simulink model "shared_control"  (R2023b)
settings: Solver=odeN  StartTime=0.0  StopTime=10.0  MaxStep=0.1  MinStep=0.01  RelTol=1e-3
values from neighbouring files (symbols this model uses):
  Bm = B    (= 4.32e-05)    [Admittance_code.m]
  D = 1    [Admittance_code.m]
  J = 2* Jm    (= 1.836e-06)    [Admittance_code.m]
  K = 0.011    [Admittance_code.m]
  Km = K    (= 0.011)    [Admittance_code.m]
  Lw = L    (= 0.00058)    [Admittance_code.m]
  M_inv = 1/J    (= 544662.309368)    [Admittance_code.m]
  Rw = R    (= 1.17)    [Admittance_code.m]
settings Model: Creator=sayeholoumi  LastModifiedBy=sayeholoumi

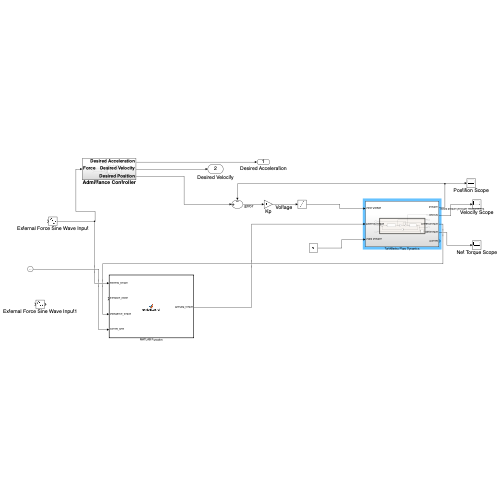
[thumbnail: Simulink's stored preview of the top-level diagram]
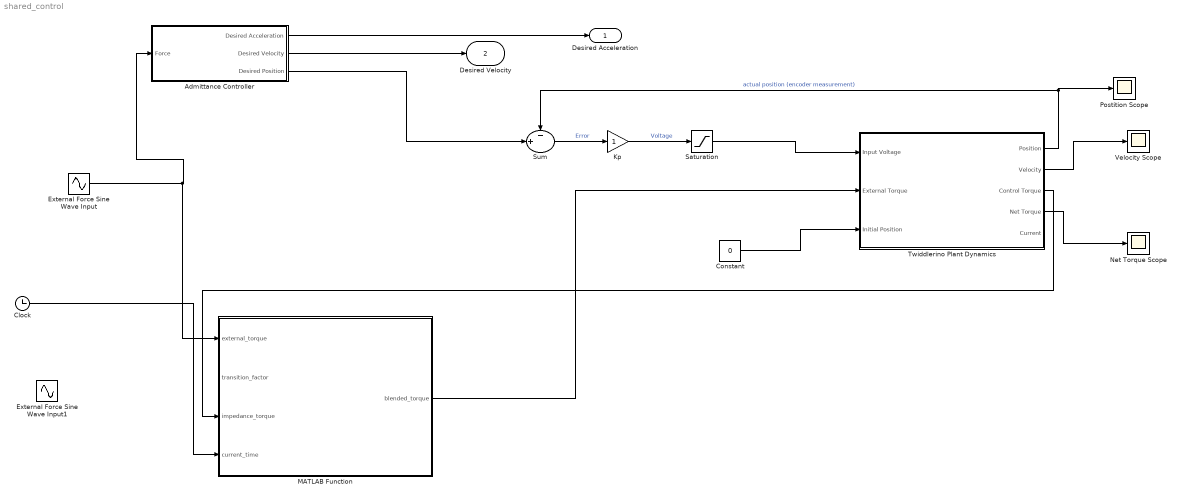
== system shared_control ==
  Admittance Controller : Subsystem
  Clock : Clock
  Constant : Constant  Value=0
  External Force Sine Wave Input : Sin  TimeSource=Use external signal  SampleTime=0
  External Force Sine Wave Input1 : Sin  TimeSource=Use external signal  SampleTime=0
  Kp : Gain
  MATLAB Function : MATLAB Function  TreatAsAtomicUnit=on
  Net Torque Scope : Scope
  Postition Scope : Scope
  Saturation : Saturate  UpperLimit=12  LowerLimit=-12
  Sum : Sum  Inputs=-+|
  Twiddlerino Plant Dynamics : Subsystem
  Velocity Scope : Scope
  Desired Acceleration : Outport
  Desired Velocity : Outport  Port=2
  wires:
  Admittance Controller/1(Desired Acceleration) -> Desired Acceleration/1
  Constant/1 -> Twiddlerino Plant Dynamics/3(Initial Position)
  Twiddlerino Plant Dynamics/2(Velocity) -> Velocity Scope/1
  Sum/1 -> Kp/1  "Error"
  Admittance Controller/3(Desired Position) -> Sum/2
  Kp/1 -> Saturation/1  "Voltage"
  Saturation/1 -> Twiddlerino Plant Dynamics/1(Input Voltage)
  Twiddlerino Plant Dynamics/4(Net Torque) -> Net Torque Scope/1
  Admittance Controller/2(Desired Velocity) -> Desired Velocity/1
  External Force Sine Wave Input/1 -> MATLAB Function/1(external_torque), Admittance Controller/1(Force)
  MATLAB Function/1(blended_torque) -> Twiddlerino Plant Dynamics/2(External Torque)
  Twiddlerino Plant Dynamics/1(Position) -> Sum/1, Postition Scope/1  "actual position (encoder measurement)"
  Twiddlerino Plant Dynamics/3(Control Torque) -> MATLAB Function/3(impedance_torque)
  Clock/1 -> MATLAB Function/4(current_time)

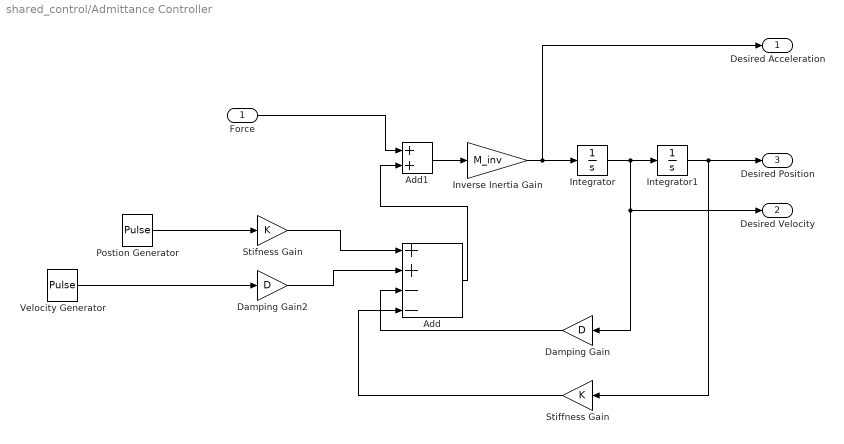
== system shared_control/Admittance Controller ==
  Force : Inport
  Add : Sum  Inputs=++--
  Add1 : Sum
  Damping Gain : Gain  Gain=D
  Damping Gain2 : Gain  Gain=D
  Integrator : Integrator
  Integrator1 : Integrator
  Inverse Inertia Gain : Gain  Gain=M_inv
  Postion Generator : DiscretePulseGenerator  PulseType=Time based  Period=10  PulseWidth=5
  "Stiffness Gain " : Gain  Gain=K
  Stifness Gain : Gain  Gain=K
  Velocity Generator : DiscretePulseGenerator  PulseType=Time based  Period=10  PulseWidth=5
  Desired Acceleration : Outport
  Desired Velocity : Outport  Port=2
  Desired Position : Outport  Port=3
  wires:
  Postion Generator/1 -> Stifness Gain/1
  Damping Gain2/1 -> Add/2
  Add/1 -> Add1/2
  Add1/1 -> Inverse Inertia Gain/1
  Damping Gain/1 -> Add/3
  Inverse Inertia Gain/1 -> Desired Acceleration/1, Integrator/1
  "Stiffness Gain "/1 -> Add/4
  Integrator1/1 -> Desired Position/1, "Stiffness Gain "/1
  Stifness Gain/1 -> Add/1
  Force/1 -> Add1/1
  Integrator/1 -> Desired Velocity/1, Damping Gain/1, Integrator1/1
  Velocity Generator/1 -> Damping Gain2/1

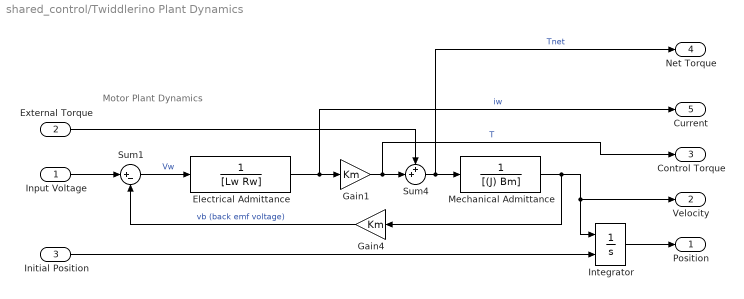
== system shared_control/Twiddlerino Plant Dynamics ==
  note: Motor Plant Dynamics
  Input Voltage : Inport
  External Torque : Inport  Port=2
  Initial Position : Inport  Port=3
  Electrical Admittance : TransferFcn  Denominator=[Lw Rw]
  Gain1 : Gain  Gain=Km
  Gain4 : Gain  Gain=Km
  Integrator : Integrator  InitialConditionSource=external
  Mechanical Admittance : TransferFcn  Denominator=[(J) Bm]
  Sum1 : Sum  Inputs=|+-
  Sum4 : Sum  Inputs=++|
  Position : Outport
  Velocity : Outport  Port=2
  Control Torque : Outport  Port=3
  Net Torque : Outport  Port=4
  Current : Outport  Port=5
  wires:
  Integrator/1 -> Position/1
  Gain1/1 -> Control Torque/1, Sum4/2  "T"
  External Torque/1 -> Sum4/1
  Electrical Admittance/1 -> Current/1, Gain1/1  "iw"
  Initial Position/1 -> Integrator/2
  Mechanical Admittance/1 -> Gain4/1, Integrator/1, Velocity/1
  Sum4/1 -> Net Torque/1, Mechanical Admittance/1  "Tnet"
  Gain4/1 -> Sum1/2  "vb (back emf voltage)"
  Input Voltage/1 -> Sum1/1
  Sum1/1 -> Electrical Admittance/1  "Vw"

== matlab function shared_control/MATLAB Function ==
  data: external_torque input; transition_factor input; impedance_torque input; blended_torque output; current_time input
function blended_torque   = unifiedControl (external_torque, transition_factor, impedance_torque, current_time)  
    if external_torque > 0
        transition_factor = -1/current_time + 1;
    else
        transition_factor = 1/current_time;
    end

    blended_torque = (1 - transition_factor) * external_torque + transition_factor * impedance_torque;
end
